simulink model "pitch_LSTM"  (R2025b)
settings: Solver=ode4  StartTime=0.0  StopTime=20  FixedStep=Ts  RelTol=1e-3
values from neighbouring files (symbols this model uses):
  den_elev = [0.1 1]    [init_pitch.m]
  nmx = no.mu_x    [testar_controladores.m]
  nmy = no.mu_y    [testar_controladores.m]
  nsx = no.sg_x    [testar_controladores.m]
  nsy = no.sg_y    [testar_controladores.m]
  num_elev = -0.1    [init_pitch.m]
  Ts = 0.01    [init_pitch.m]
  x0_din = [0; 0]    [init_pitch.m]    (also in testar_controladores.m = [Cdin; Cdin*Adin] \ [deg2rad(theta0_deg); 0])
undefined symbols (not defined in the file or in its folder): Adin, Bdin, Cdin, Ddin
libraries: deeplib x1
settings Model: Creator=kauemartinsdesouza  LastModifiedBy=kauemartinsdesouza

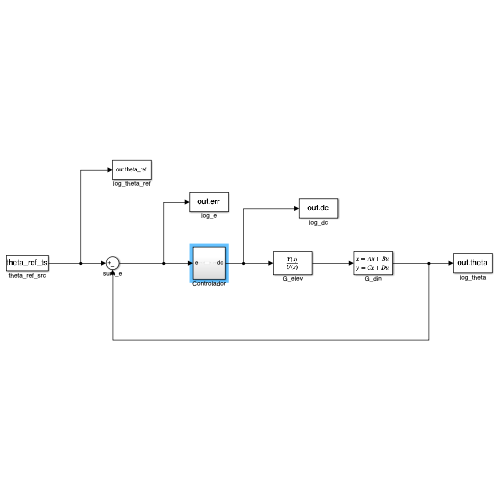
[thumbnail: Simulink's stored preview of the top-level diagram]
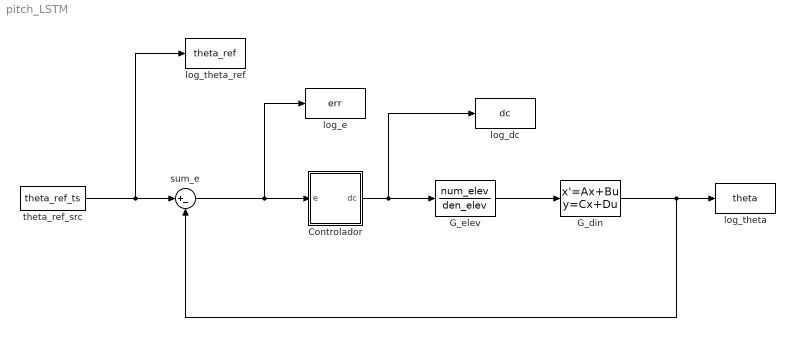
== system pitch_LSTM ==
  Controlador : Subsystem
  G_din : StateSpace  A=Adin  B=Bdin  C=Cdin  D=Ddin  InitialCondition=x0_din
  G_elev : TransferFcn  Numerator=num_elev  Denominator=den_elev
  log_dc : ToWorkspace  VariableName=dc  SaveFormat=Timeseries  SampleTime=-1
  log_e : ToWorkspace  VariableName=err  SaveFormat=Timeseries  SampleTime=-1
  log_theta : ToWorkspace  VariableName=theta  SaveFormat=Timeseries  SampleTime=-1
  log_theta_ref : ToWorkspace  VariableName=theta_ref  SaveFormat=Timeseries  SampleTime=-1
  sum_e : Sum  Inputs=|+-
  theta_ref_src : FromWorkspace  VariableName=theta_ref_ts  SampleTime=Ts  Interpolate=off  OutputAfterFinalValue=Holding final value
  wires:
  theta_ref_src/1 -> log_theta_ref/1, sum_e/1
  sum_e/1 -> Controlador/1(e), log_e/1
  G_elev/1 -> G_din/1
  G_din/1 -> log_theta/1, sum_e/2
  Controlador/1(dc) -> log_dc/1, G_elev/1

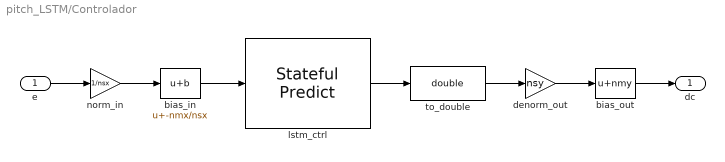
== system pitch_LSTM/Controlador ==
  e : Inport
  bias_in : Bias  Bias=-nmx/nsx
  bias_out : Bias  Bias=nmy
  denorm_out : Gain  Gain=nsy
  lstm_ctrl : deeplib/Stateful Predict  Network=Network from MAT-file  NetworkFunction=net  NetworkFilePath=net_pitch.mat  InputDataFormats={'sequenceinput', 'TCB';}  SampleTime=Ts  ForceInterpretedSim=on  EnableDLNetwork=on  LastKnownNetworkFilePath='net_pitch.mat'  LastKnownNetworkTimeStamp=740150.606435185181908309459686279296875
  norm_in : Gain  Gain=1/nsx
  to_double : DataTypeConversion  OutDataTypeStr=double  SaturateOnIntegerOverflow=off  RndMeth=Floor
  dc : Outport
  wires:
  e/1 -> norm_in/1
  norm_in/1 -> bias_in/1
  bias_in/1 -> lstm_ctrl/1
  lstm_ctrl/1 -> to_double/1
  to_double/1 -> denorm_out/1
  denorm_out/1 -> bias_out/1
  bias_out/1 -> dc/1
